simulink model "StateSpace"  (R2021a)
settings: Solver=VariableStepAuto  StartTime=0.0  StopTime=500  RelTol=1e-3
values from neighbouring files (symbols this model uses):
  C = [1,0,0]    [main.m]
  D = 0    [main.m]
  G = tf(ExpFun(tf('s')))    [main.m]
undefined symbols (not defined in the file or in its folder): H, K_deadbeat, L, Ts
settings Model: Creator=arman  LastModifiedBy=arman

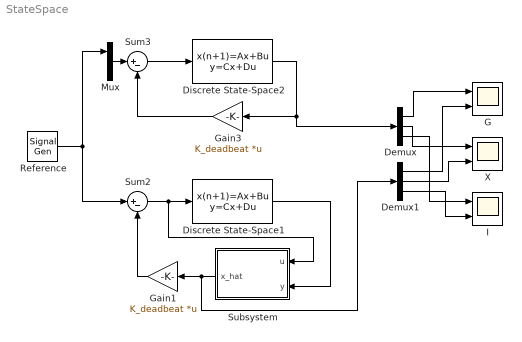
== system StateSpace ==
  Demux : Demux  Outputs=3
  Demux1 : Demux  Outputs=3
  Discrete State-Space1 : DiscreteStateSpace  A=G  B=H  C=C  D=D  SampleTime=Ts
  Discrete State-Space2 : DiscreteStateSpace  A=G  B=[H zeros(3,2)]  C=eye(3)  D=zeros(3)  SampleTime=Ts
  G : Scope  NumInputPorts=2
  Gain1 : Gain  Gain=K_deadbeat  Multiplication=Matrix(K*u)
  Gain3 : Gain  Gain=K_deadbeat  Multiplication=Matrix(K*u)
  I : Scope  NumInputPorts=2
  Mux : Mux  Inputs=3
  Reference : SignalGenerator  Frequency=0.005
  Subsystem : Subsystem
  Sum2 : Sum  Inputs=|+-
  Sum3 : Sum  Inputs=|+-
  X : Scope  NumInputPorts=2
  wires:
  Sum2/1 -> Subsystem/1(u), Discrete State-Space1/1
  Gain1/1 -> Sum2/2
  Subsystem/1(x_hat) -> Gain1/1, Demux1/1
  Discrete State-Space1/1 -> Subsystem/2(y)
  Gain3/1 -> Sum3/2
  Sum3/1 -> Discrete State-Space2/1
  Reference/1 -> Mux/1, Sum2/1
  Mux/1 -> Sum3/1
  Discrete State-Space2/1 -> Gain3/1, Demux/1
  Demux/1 -> G/1
  Demux1/1 -> G/2
  Demux/2 -> X/1
  Demux1/2 -> X/2
  Demux/3 -> I/1
  Demux1/3 -> I/2

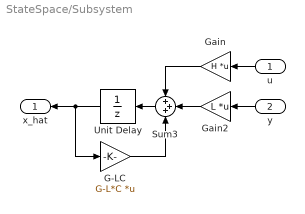
== system StateSpace/Subsystem ==
  u : Inport
  y : Inport  Port=2
  G-LC : Gain  Gain=G-L*C  Multiplication=Matrix(K*u)
  Gain : Gain  Gain=H  Multiplication=Matrix(K*u)
  Gain2 : Gain  Gain=L  Multiplication=Matrix(K*u)
  Sum3 : Sum  Inputs=+++
  Unit Delay : UnitDelay  SampleTime=-1  HasFrameUpgradeWarning=on
  x_hat : Outport
  wires:
  G-LC/1 -> Sum3/3
  u/1 -> Gain/1
  Sum3/1 -> Unit Delay/1
  Unit Delay/1 -> x_hat/1, G-LC/1
  Gain/1 -> Sum3/1
  y/1 -> Gain2/1
  Gain2/1 -> Sum3/2
